simulink model "generic_src"  (Simulink 10.3)
settings: Solver=ode45  StartTime=0.0  StopTime=inf  RelTol=1e-3  EnableMultiTasking=on
undefined symbols (not defined in the file or in its folder): Area_Front, Area_Rear, ay_max_off, ay_max_on, ay_per_mu_max_off, ay_per_mu_max_on, Brake_ratio, brake_valve_ctrl_kP, cat1mode1_higher, cat1mode1_lower, cat1mode2_higher, cat1mode2_lower, cat1mode3_higher, cat1mode3_lower, cat2mode1_higher, cat2mode1_lower, cat2mode2_higher, cat2mode2_lower, cat2mode3_higher, cat2mode3_lower, delta_vel, diff_lock_fac, diff_lock_off, diff_lock_on, ESP_ctrl_kD, ESP_ctrl_kI, ESP_ctrl_kP, ESP_ctrl_restore_kI, ESP_min_throttle_fac, f_ax, f_slip, g, higherlimit_highvel, higherlimit_lowvel, highervel_fac, highervelocity_fac, InitialConditionForIntegrator, limit_acc, limit_selectlow, limit_starting, limit_vdiff, locktime_throttle, lowerlimit_highvel, lowerlimit_lowvel, lowervel_fac, lowervelocity_fac, min_throttle, MPS2KMPH, MSR_ctrl_kD, MSR_ctrl_kI, MSR_ctrl_kP, MSR_min_throttle_fac, PID_kP_sideslip, PID_kP_yawrate, RADpS2RpM, rBrake, RpM2RADpS, SH_SL_switch, sideslip_vel_corr, sidesplip_deviation_max ... (+35)
libraries: CarMaker4SL x137, simulink x57, simulink_extras x6
(part 3 of 12)

== system generic_src/CarMaker/IPG Vehicle/PowerTrain/PTControl Example/PTC GearBoxOut ==
  GearBoxOut GearNoTrg : Inport
  Bus Assignment1 : BusAssignment  AssignedSignals=PTC GearboxOut0 GearNoTrg
  BusCreator : BusCreator  Inputs=12
  CreateBus PTC GearboxOut0 : Subsystem
  CreateBus PTC GearboxOut1 : Subsystem
  CreateBus PTC GearboxOut10 : Subsystem
  CreateBus PTC GearboxOut11 : Subsystem
  CreateBus PTC GearboxOut2 : Subsystem
  CreateBus PTC GearboxOut3 : Subsystem
  CreateBus PTC GearboxOut4 : Subsystem
  CreateBus PTC GearboxOut5 : Subsystem
  CreateBus PTC GearboxOut6 : Subsystem
  CreateBus PTC GearboxOut7 : Subsystem
  CreateBus PTC GearboxOut8 : Subsystem
  CreateBus PTC GearboxOut9 : Subsystem
  Ground PTC GearboxOut{0..11} (12 alike) : Ground
  PTC GearboxOut : Outport
  wires:
  GearBoxOut GearNoTrg/1 -> Bus Assignment1/2
  Ground PTC GearboxOut0/1 -> CreateBus PTC GearboxOut0/1(In)
  CreateBus PTC GearboxOut0/1(Out) -> Bus Assignment1/1
  Ground PTC GearboxOut3/1 -> CreateBus PTC GearboxOut3/1(In)
  Ground PTC GearboxOut2/1 -> CreateBus PTC GearboxOut2/1(In)
  Ground PTC GearboxOut1/1 -> CreateBus PTC GearboxOut1/1(In)
  Ground PTC GearboxOut4/1 -> CreateBus PTC GearboxOut4/1(In)
  Ground PTC GearboxOut5/1 -> CreateBus PTC GearboxOut5/1(In)
  Ground PTC GearboxOut6/1 -> CreateBus PTC GearboxOut6/1(In)
  Ground PTC GearboxOut7/1 -> CreateBus PTC GearboxOut7/1(In)
  Ground PTC GearboxOut8/1 -> CreateBus PTC GearboxOut8/1(In)
  Ground PTC GearboxOut9/1 -> CreateBus PTC GearboxOut9/1(In)
  Ground PTC GearboxOut10/1 -> CreateBus PTC GearboxOut10/1(In)
  Ground PTC GearboxOut11/1 -> CreateBus PTC GearboxOut11/1(In)
  Bus Assignment1/1 -> BusCreator/1  "PTC GearBoxOut0"
  CreateBus PTC GearboxOut1/1(Out) -> BusCreator/2  "PTC GearBoxOut1"
  CreateBus PTC GearboxOut2/1(Out) -> BusCreator/3  "PTC GearBoxOut2"
  CreateBus PTC GearboxOut3/1(Out) -> BusCreator/4  "PTC GearBoxOut3"
  CreateBus PTC GearboxOut4/1(Out) -> BusCreator/5  "PTC GearBoxOut4"
  CreateBus PTC GearboxOut5/1(Out) -> BusCreator/6  "PTC GearBoxOut5"
  CreateBus PTC GearboxOut6/1(Out) -> BusCreator/7  "PTC GearBoxOut6"
  CreateBus PTC GearboxOut7/1(Out) -> BusCreator/8  "PTC GearBoxOut7"
  CreateBus PTC GearboxOut8/1(Out) -> BusCreator/9  "PTC GearBoxOut8"
  CreateBus PTC GearboxOut9/1(Out) -> BusCreator/10  "PTC GearBoxOut9"
  CreateBus PTC GearboxOut10/1(Out) -> BusCreator/11  "PTC GearBoxOut10"
  CreateBus PTC GearboxOut11/1(Out) -> BusCreator/12  "PTC GearBoxOut11"
  BusCreator/1 -> PTC GearboxOut/1  "PTC GearboxOut"

== system generic_src/CarMaker/IPG Vehicle/PowerTrain/PTControl Example/PTC MotorOut ==
  BusCreator : BusCreator  Inputs=12
  CreateBus PTC MotorOut0 : Subsystem
  CreateBus PTC MotorOut1 : Subsystem
  CreateBus PTC MotorOut10 : Subsystem
  CreateBus PTC MotorOut11 : Subsystem
  CreateBus PTC MotorOut2 : Subsystem
  CreateBus PTC MotorOut3 : Subsystem
  CreateBus PTC MotorOut4 : Subsystem
  CreateBus PTC MotorOut5 : Subsystem
  CreateBus PTC MotorOut6 : Subsystem
  CreateBus PTC MotorOut7 : Subsystem
  CreateBus PTC MotorOut8 : Subsystem
  CreateBus PTC MotorOut9 : Subsystem
  Ground PTC MotorOut{0..11} (12 alike) : Ground
  PTC MotorOut : Outport
  wires:
  CreateBus PTC MotorOut0/1(Out) -> BusCreator/1  "PTC MotorOut0"
  Ground PTC MotorOut0/1 -> CreateBus PTC MotorOut0/1(In)
  Ground PTC MotorOut3/1 -> CreateBus PTC MotorOut3/1(In)
  Ground PTC MotorOut1/1 -> CreateBus PTC MotorOut1/1(In)
  CreateBus PTC MotorOut1/1(Out) -> BusCreator/2  "PTC MotorOut1"
  Ground PTC MotorOut4/1 -> CreateBus PTC MotorOut4/1(In)
  Ground PTC MotorOut2/1 -> CreateBus PTC MotorOut2/1(In)
  CreateBus PTC MotorOut2/1(Out) -> BusCreator/3  "PTC MotorOut2"
  Ground PTC MotorOut5/1 -> CreateBus PTC MotorOut5/1(In)
  Ground PTC MotorOut6/1 -> CreateBus PTC MotorOut6/1(In)
  Ground PTC MotorOut7/1 -> CreateBus PTC MotorOut7/1(In)
  Ground PTC MotorOut8/1 -> CreateBus PTC MotorOut8/1(In)
  Ground PTC MotorOut9/1 -> CreateBus PTC MotorOut9/1(In)
  Ground PTC MotorOut10/1 -> CreateBus PTC MotorOut10/1(In)
  Ground PTC MotorOut11/1 -> CreateBus PTC MotorOut11/1(In)
  CreateBus PTC MotorOut4/1(Out) -> BusCreator/5  "PTC MotorOut4"
  CreateBus PTC MotorOut5/1(Out) -> BusCreator/6  "PTC MotorOut5"
  CreateBus PTC MotorOut6/1(Out) -> BusCreator/7  "PTC MotorOut6"
  CreateBus PTC MotorOut7/1(Out) -> BusCreator/8  "PTC MotorOut7"
  CreateBus PTC MotorOut8/1(Out) -> BusCreator/9  "PTC MotorOut8"
  CreateBus PTC MotorOut9/1(Out) -> BusCreator/10  "PTC MotorOut9"
  CreateBus PTC MotorOut10/1(Out) -> BusCreator/11  "PTC MotorOut10"
  CreateBus PTC MotorOut11/1(Out) -> BusCreator/12  "PTC MotorOut11"
  CreateBus PTC MotorOut3/1(Out) -> BusCreator/4  "PTC MotorOut3"
  BusCreator/1 -> PTC MotorOut/1  "CreateBus PTC MotorOut"

== system generic_src/CarMaker/IPG Vehicle/PowerTrain/PTControl Example/PTControl Example ==
  note: Minimalistic PTControl example model, that only works with
      | the 'Generic' powertrain and the 'Manual' gearbox.
  EngineIn : Inport
  VhclCtrl.PT : Inport  Port=2
  Bus Selector : BusSelector  OutputSignals=VhclCtrl Key,VhclCtrl Gas,VhclCtrl Clutch,VhclCtrl GearNo
  Bus Selector1 : BusSelector  OutputSignals=PTC EngineIn.PTC EngineIn Engine_on
  Engine : Subsystem
  ISG : Subsystem
  PTC : Subsystem
  PTC MiscOut : Outport  VectorParamsAs1DForOutWhenUnconnected=off
  EngineOut : Outport  Port=2  VectorParamsAs1DForOutWhenUnconnected=off
  ISGOut : Outport  Port=3  VectorParamsAs1DForOutWhenUnconnected=off
  ClutchOut Pos : Outport  Port=4  VectorParamsAs1DForOutWhenUnconnected=off
  GearBoxOut GearNoTrg : Outport  Port=5  VectorParamsAs1DForOutWhenUnconnected=off
  wires:
  VhclCtrl.PT/1 -> Bus Selector/1
  EngineIn/1 -> Bus Selector1/1
  Engine/1(EngineOut) -> EngineOut/1
  Bus Selector1/1 -> Engine/2(Engine_on), PTC/2(Engine_on)  "<PTC EngineIn Engine_on>"
  Bus Selector/2 -> Engine/1(Gas)  "<VhclCtrl Gas>"
  ISG/1(ISGOut) -> ISGOut/1
  PTC/1(PTC MiscOut) -> PTC MiscOut/1
  Bus Selector/4 -> GearBoxOut GearNoTrg/1  "<VhclCtrl GearNo>"
  Bus Selector/3 -> ClutchOut Pos/1  "<VhclCtrl Clutch>"
  Bus Selector/1 -> PTC/1(Key), ISG/1(Key)  "<VhclCtrl Key>"

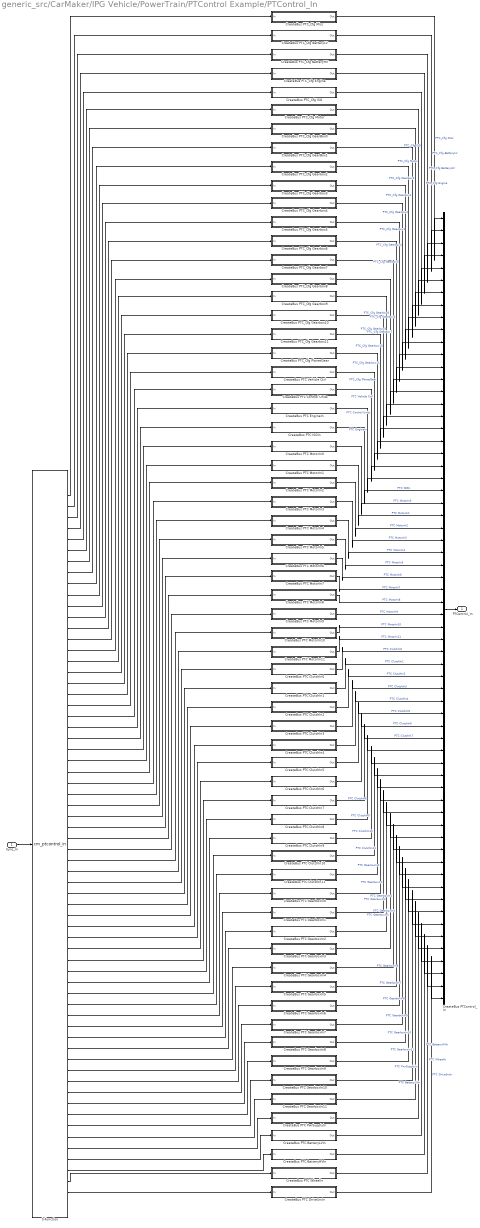
== system generic_src/CarMaker/IPG Vehicle/PowerTrain/PTControl Example/PTControl_In ==
  Sync_In : Inport
  CreateBus PTC BatteryHVIn : Subsystem
  CreateBus PTC BatteryLVIn : Subsystem
  CreateBus PTC ClutchIn0 : Subsystem
  CreateBus PTC ClutchIn1 : Subsystem
  CreateBus PTC ClutchIn10 : Subsystem
  CreateBus PTC ClutchIn11 : Subsystem
  CreateBus PTC ClutchIn2 : Subsystem
  CreateBus PTC ClutchIn3 : Subsystem
  CreateBus PTC ClutchIn4 : Subsystem
  CreateBus PTC ClutchIn5 : Subsystem
  CreateBus PTC ClutchIn6 : Subsystem
  CreateBus PTC ClutchIn7 : Subsystem
  CreateBus PTC ClutchIn8 : Subsystem
  CreateBus PTC ClutchIn9 : Subsystem
  CreateBus PTC Control Units : Subsystem
  CreateBus PTC DriveSrcIn : Subsystem
  CreateBus PTC EngineIn : Subsystem
  CreateBus PTC GearboxIn0 : Subsystem
  CreateBus PTC GearboxIn1 : Subsystem
  CreateBus PTC GearboxIn10 : Subsystem
  CreateBus PTC GearboxIn11 : Subsystem
  CreateBus PTC GearboxIn2 : Subsystem
  CreateBus PTC GearboxIn3 : Subsystem
  CreateBus PTC GearboxIn4 : Subsystem
  CreateBus PTC GearboxIn5 : Subsystem
  CreateBus PTC GearboxIn6 : Subsystem
  CreateBus PTC GearboxIn7 : Subsystem
  CreateBus PTC GearboxIn8 : Subsystem
  CreateBus PTC GearboxIn9 : Subsystem
  CreateBus PTC ISGIn : Subsystem
  CreateBus PTC MotorIn0 : Subsystem
  CreateBus PTC MotorIn1 : Subsystem
  CreateBus PTC MotorIn10 : Subsystem
  CreateBus PTC MotorIn11 : Subsystem
  CreateBus PTC MotorIn2 : Subsystem
  CreateBus PTC MotorIn3 : Subsystem
  CreateBus PTC MotorIn4 : Subsystem
  CreateBus PTC MotorIn5 : Subsystem
  CreateBus PTC MotorIn6 : Subsystem
  CreateBus PTC MotorIn7 : Subsystem
  CreateBus PTC MotorIn8 : Subsystem
  CreateBus PTC MotorIn9 : Subsystem
  CreateBus PTC PwrSupplyIn : Subsystem
  CreateBus PTC Vehicle Ctrl : Subsystem
  CreateBus PTC WheelIn : Subsystem
  CreateBus PTC_Cfg BatteryHV : Subsystem
  CreateBus PTC_Cfg BatteryLV : Subsystem
  CreateBus PTC_Cfg Engine : Subsystem
  CreateBus PTC_Cfg GearBox0 : Subsystem
  CreateBus PTC_Cfg GearBox1 : Subsystem
  CreateBus PTC_Cfg Gearbox10 : Subsystem
  CreateBus PTC_Cfg Gearbox11 : Subsystem
  CreateBus PTC_Cfg Gearbox2 : Subsystem
  CreateBus PTC_Cfg Gearbox3 : Subsystem
  CreateBus PTC_Cfg Gearbox4 : Subsystem
  CreateBus PTC_Cfg Gearbox5 : Subsystem
  CreateBus PTC_Cfg Gearbox6 : Subsystem
  CreateBus PTC_Cfg Gearbox7 : Subsystem
  CreateBus PTC_Cfg Gearbox8 : Subsystem
  CreateBus PTC_Cfg Gearbox9 : Subsystem
  CreateBus PTC_Cfg ISG : Subsystem
  CreateBus PTC_Cfg Misc : Subsystem
  CreateBus PTC_Cfg Motor : Subsystem
  CreateBus PTC_Cfg PlanetGear : Subsystem
  CreateBus PTControl_In : BusCreator  Inputs=64
  S-Function : S-Function  FunctionName=cm_ptcontrol_in  SFunctionDeploymentMode=off  EnableBusSupport=off
  PTControl_In : Outport  VectorParamsAs1DForOutWhenUnconnected=off
  wires:
  CreateBus PTControl_In/1 -> PTControl_In/1
  Sync_In/1 -> S-Function/1
  S-Function/2 -> CreateBus PTC_Cfg BatteryLV/1(In)
  CreateBus PTC_Cfg Misc/1(Out) -> CreateBus PTControl_In/1  "PTC_Cfg Misc"
  S-Function/1 -> CreateBus PTC_Cfg Misc/1(In)
  CreateBus PTC_Cfg Motor/1(Out) -> CreateBus PTControl_In/6  "PTC_Cfg Motor"
  CreateBus PTC_Cfg Gearbox2/1(Out) -> CreateBus PTControl_In/9  "PTC_Cfg Gearbox2"
  S-Function/4 -> CreateBus PTC_Cfg Engine/1(In)
  S-Function/3 -> CreateBus PTC_Cfg BatteryHV/1(In)
  S-Function/7 -> CreateBus PTC_Cfg GearBox0/1(In)
  S-Function/14 -> CreateBus PTC_Cfg Gearbox7/1(In)
  S-Function/15 -> CreateBus PTC_Cfg Gearbox8/1(In)
  S-Function/17 -> CreateBus PTC_Cfg Gearbox10/1(In)
  S-Function/18 -> CreateBus PTC_Cfg Gearbox11/1(In)
  CreateBus PTC_Cfg GearBox1/1(Out) -> CreateBus PTControl_In/8  "PTC_Cfg Gearbox1"
  CreateBus PTC_Cfg Gearbox4/1(Out) -> CreateBus PTControl_In/11  "PTC_Cfg Gearbox4"
  CreateBus PTC_Cfg Gearbox5/1(Out) -> CreateBus PTControl_In/12  "PTC_Cfg Gearbox5"
  CreateBus PTC_Cfg Gearbox6/1(Out) -> CreateBus PTControl_In/13  "PTC_Cfg Gearbox6"
  CreateBus PTC_Cfg Gearbox7/1(Out) -> CreateBus PTControl_In/14  "PTC_Cfg Gearbox7"
  CreateBus PTC GearboxIn6/1(Out) -> CreateBus PTControl_In/54  "PTC GearboxIn6"
  CreateBus PTC ClutchIn6/1(Out) -> CreateBus PTControl_In/42  "PTC ClutchIn6"
  CreateBus PTC GearboxIn5/1(Out) -> CreateBus PTControl_In/53  "PTC GearboxIn5"
  CreateBus PTC GearboxIn9/1(Out) -> CreateBus PTControl_In/57  "PTC GearboxIn9"
  CreateBus PTC ClutchIn8/1(Out) -> CreateBus PTControl_In/44  "PTC ClutchIn8"
  S-Function/32 -> CreateBus PTC MotorIn8/1(In)
  CreateBus PTC MotorIn0/1(Out) -> CreateBus PTControl_In/24  "PTC MotorIn0"
  S-Function/8 -> CreateBus PTC_Cfg GearBox1/1(In)
  S-Function/46 -> CreateBus PTC ClutchIn10/1(In)
  S-Function/61 -> CreateBus PTC BatteryLVIn/1(In)
  S-Function/11 -> CreateBus PTC_Cfg Gearbox4/1(In)
  S-Function/37 -> CreateBus PTC ClutchIn1/1(In)
  S-Function/50 -> CreateBus PTC GearboxIn2/1(In)
  CreateBus PTC WheelIn/1(Out) -> CreateBus PTControl_In/63  "PTC WheelIn"
  S-Function/24 -> CreateBus PTC MotorIn0/1(In)
  CreateBus PTC_Cfg Gearbox3/1(Out) -> CreateBus PTControl_In/10  "PTC_Cfg Gearbox3"
  S-Function/51 -> CreateBus PTC GearboxIn3/1(In)
  S-Function/56 -> CreateBus PTC GearboxIn8/1(In)
  CreateBus PTC GearboxIn3/1(Out) -> CreateBus PTControl_In/51  "PTC GearboxIn3"
  CreateBus PTC MotorIn1/1(Out) -> CreateBus PTControl_In/25  "PTC MotorIn1"
  S-Function/10 -> CreateBus PTC_Cfg Gearbox3/1(In)
  CreateBus PTC DriveSrcIn/1(Out) -> CreateBus PTControl_In/64  "PTC DriveSrcIn"
  CreateBus PTC ISGIn/1(Out) -> CreateBus PTControl_In/23  "PTC ISGIn"
  CreateBus PTC ClutchIn11/1(Out) -> CreateBus PTControl_In/47  "PTC ClutchIn11"
  S-Function/20 -> CreateBus PTC Vehicle Ctrl/1(In)
  S-Function/47 -> CreateBus PTC ClutchIn11/1(In)
  S-Function/64 -> CreateBus PTC DriveSrcIn/1(In)
  CreateBus PTC ClutchIn10/1(Out) -> CreateBus PTControl_In/46  "PTC ClutchIn10"
  CreateBus PTC GearboxIn2/1(Out) -> CreateBus PTControl_In/50  "PTC GearboxIn2"
  CreateBus PTC GearboxIn0/1(Out) -> CreateBus PTControl_In/48  "PTC GearboxIn0"
  S-Function/16 -> CreateBus PTC_Cfg Gearbox9/1(In)
  S-Function/25 -> CreateBus PTC MotorIn1/1(In)
  S-Function/63 -> CreateBus PTC WheelIn/1(In)
  CreateBus PTC GearboxIn1/1(Out) -> CreateBus PTControl_In/49  "PTC GearboxIn1"
  S-Function/33 -> CreateBus PTC MotorIn9/1(In)
  CreateBus PTC BatteryLVIn/1(Out) -> CreateBus PTControl_In/61  "PTC BatteryLVIn"
  S-Function/58 -> CreateBus PTC GearboxIn10/1(In)
  S-Function/41 -> CreateBus PTC ClutchIn5/1(In)
  S-Function/5 -> CreateBus PTC_Cfg ISG/1(In)
  S-Function/44 -> CreateBus PTC ClutchIn8/1(In)
  S-Function/45 -> CreateBus PTC ClutchIn9/1(In)
  CreateBus PTC GearboxIn11/1(Out) -> CreateBus PTControl_In/59  "PTC GearboxIn11"
  S-Function/9 -> CreateBus PTC_Cfg Gearbox2/1(In)
  S-Function/35 -> CreateBus PTC MotorIn11/1(In)
  S-Function/19 -> CreateBus PTC_Cfg PlanetGear/1(In)
  CreateBus PTC GearboxIn8/1(Out) -> CreateBus PTControl_In/56  "PTC GearboxIn8"
  S-Function/36 -> CreateBus PTC ClutchIn0/1(In)
  S-Function/53 -> CreateBus PTC GearboxIn5/1(In)
  CreateBus PTC GearboxIn10/1(Out) -> CreateBus PTControl_In/58  "PTC GearboxIn10"
  S-Function/6 -> CreateBus PTC_Cfg Motor/1(In)
  CreateBus PTC PwrSupplyIn/1(Out) -> CreateBus PTControl_In/60  "PTC PwrSupplyIn"
  S-Function/43 -> CreateBus PTC ClutchIn7/1(In)
  CreateBus PTC_Cfg BatteryLV/1(Out) -> CreateBus PTControl_In/2  "PTC_Cfg BatteryLV"
  CreateBus PTC ClutchIn1/1(Out) -> CreateBus PTControl_In/37  "PTC ClutchIn1"
  S-Function/26 -> CreateBus PTC MotorIn2/1(In)
  CreateBus PTC_Cfg PlanetGear/1(Out) -> CreateBus PTControl_In/19  "PTC_Cfg PlanetGear"
  CreateBus PTC_Cfg Gearbox10/1(Out) -> CreateBus PTControl_In/17  "PTC_Cfg Gearbox10"
  CreateBus PTC ClutchIn7/1(Out) -> CreateBus PTControl_In/43  "PTC ClutchIn7"
  S-Function/54 -> CreateBus PTC GearboxIn6/1(In)
  S-Function/29 -> CreateBus PTC MotorIn5/1(In)
  CreateBus PTC_Cfg BatteryHV/1(Out) -> CreateBus PTControl_In/3  "PTC_Cfg BatteryHV"
  S-Function/13 -> CreateBus PTC_Cfg Gearbox6/1(In)
  CreateBus PTC ClutchIn9/1(Out) -> CreateBus PTControl_In/45  "PTC ClutchIn9"
  CreateBus PTC GearboxIn4/1(Out) -> CreateBus PTControl_In/52  "PTC GearboxIn4"
  S-Function/57 -> CreateBus PTC GearboxIn9/1(In)
  CreateBus PTC GearboxIn7/1(Out) -> CreateBus PTControl_In/55  "PTC GearboxIn7"
  S-Function/60 -> CreateBus PTC PwrSupplyIn/1(In)
  CreateBus PTC BatteryHVIn/1(Out) -> CreateBus PTControl_In/62  "PTC BatteryHVIn"
  S-Function/49 -> CreateBus PTC GearboxIn1/1(In)
  S-Function/55 -> CreateBus PTC GearboxIn7/1(In)
  S-Function/21 -> CreateBus PTC Control Units/1(In)
  CreateBus PTC ClutchIn5/1(Out) -> CreateBus PTControl_In/41  "PTC ClutchIn5"
  CreateBus PTC ClutchIn4/1(Out) -> CreateBus PTControl_In/40  "PTC ClutchIn4"
  S-Function/38 -> CreateBus PTC ClutchIn2/1(In)
  CreateBus PTC Control Units/1(Out) -> CreateBus PTControl_In/21  "PTC Control Units"
  S-Function/40 -> CreateBus PTC ClutchIn4/1(In)
  CreateBus PTC MotorIn11/1(Out) -> CreateBus PTControl_In/35  "PTC MotorIn11"
  CreateBus PTC ClutchIn3/1(Out) -> CreateBus PTControl_In/39  "PTC ClutchIn3"
  S-Function/39 -> CreateBus PTC ClutchIn3/1(In)
  CreateBus PTC MotorIn2/1(Out) -> CreateBus PTControl_In/26  "PTC MotorIn2"
  CreateBus PTC ClutchIn2/1(Out) -> CreateBus PTControl_In/38  "PTC ClutchIn2"
  CreateBus PTC_Cfg ISG/1(Out) -> CreateBus PTControl_In/5  "PTC_Cfg ISG"
  CreateBus PTC ClutchIn0/1(Out) -> CreateBus PTControl_In/36  "PTC ClutchIn0"
  S-Function/52 -> CreateBus PTC GearboxIn4/1(In)
  CreateBus PTC EngineIn/1(Out) -> CreateBus PTControl_In/22  "PTC EngineIn"
  CreateBus PTC_Cfg GearBox0/1(Out) -> CreateBus PTControl_In/7  "PTC_Cfg Gearbox0"
  S-Function/42 -> CreateBus PTC ClutchIn6/1(In)
  S-Function/34 -> CreateBus PTC MotorIn10/1(In)
  CreateBus PTC MotorIn9/1(Out) -> CreateBus PTControl_In/33  "PTC MotorIn9"
  S-Function/30 -> CreateBus PTC MotorIn6/1(In)
  S-Function/12 -> CreateBus PTC_Cfg Gearbox5/1(In)
  CreateBus PTC MotorIn8/1(Out) -> CreateBus PTControl_In/32  "PTC MotorIn8"
  CreateBus PTC MotorIn7/1(Out) -> CreateBus PTControl_In/31  "PTC MotorIn7"
  S-Function/31 -> CreateBus PTC MotorIn7/1(In)
  CreateBus PTC MotorIn6/1(Out) -> CreateBus PTControl_In/30  "PTC MotorIn6"
  CreateBus PTC MotorIn4/1(Out) -> CreateBus PTControl_In/28  "PTC MotorIn4"
  S-Function/62 -> CreateBus PTC BatteryHVIn/1(In)
  S-Function/27 -> CreateBus PTC MotorIn3/1(In)
  S-Function/28 -> CreateBus PTC MotorIn4/1(In)
  CreateBus PTC MotorIn5/1(Out) -> CreateBus PTControl_In/29  "PTC MotorIn5"
  CreateBus PTC MotorIn3/1(Out) -> CreateBus PTControl_In/27  "PTC MotorIn3"
  S-Function/23 -> CreateBus PTC ISGIn/1(In)
  S-Function/22 -> CreateBus PTC EngineIn/1(In)
  CreateBus PTC_Cfg Engine/1(Out) -> CreateBus PTControl_In/4  "PTC_Cfg Engine"
  S-Function/48 -> CreateBus PTC GearboxIn0/1(In)
  S-Function/59 -> CreateBus PTC GearboxIn11/1(In)
  CreateBus PTC Vehicle Ctrl/1(Out) -> CreateBus PTControl_In/20  "PTC Vehicle Ctrl"
  CreateBus PTC MotorIn10/1(Out) -> CreateBus PTControl_In/34  "PTC MotorIn10"
  CreateBus PTC_Cfg Gearbox11/1(Out) -> CreateBus PTControl_In/18  "PTC_Cfg Gearbox11"
  CreateBus PTC_Cfg Gearbox9/1(Out) -> CreateBus PTControl_In/16  "PTC_Cfg Gearbox9"
  CreateBus PTC_Cfg Gearbox8/1(Out) -> CreateBus PTControl_In/15  "PTC_Cfg Gearbox8"

== system generic_src/CarMaker/IPG Vehicle/PowerTrain/PTControl Example/PTControl_Out ==
  PTC MiscOut : Inport
  PTC EngineOut : Inport  Port=2
  PTC ISGOut : Inport  Port=3
  PTC MotorOut : Inport  Port=4
  PTC ClutchOut : Inport  Port=5
  PTC GearboxOut : Inport  Port=6
  PTC PwrSupplyOut : Inport  Port=7
  PTC BattLV_Out : Inport  Port=8
  PTC BattHV_Out : Inport  Port=9
  PTC WheelOut : Inport  Port=10
  Bus Selector1 : BusSelector  OutputSignals=PTC MotorOut0,PTC MotorOut1,PTC MotorOut2,PTC MotorOut3,PTC MotorOut4,PTC MotorOut5,PTC MotorOut6,PTC MotorOut7,PTC MotorOut8,PTC MotorOut9,PTC MotorOut10,PTC MotorOut11
  Bus Selector2 : BusSelector  OutputSignals=PTC ClutchOut0,PTC ClutchOut1,PTC ClutchOut2,PTC ClutchOut3,PTC ClutchOut4,PTC ClutchOut5,PTC ClutchOut6,PTC ClutchOut7,PTC ClutchOut8,PTC ClutchOut9,PTC ClutchOut10,PTC ClutchOut11
  Bus Selector3 : BusSelector  OutputSignals=PTC GearBoxOut0,PTC GearBoxOut1,PTC GearBoxOut2,PTC GearBoxOut3,PTC GearBoxOut4,PTC GearBoxOut5,PTC GearBoxOut6,PTC GearBoxOut7,PTC GearBoxOut8,PTC GearBoxOut9,PTC GearBoxOut10,PTC GearBoxOut11
  PTControl_Out : S-Function  FunctionName=cm_ptcontrol_out  SFunctionDeploymentMode=off  EnableBusSupport=off
  wires:
  PTC MotorOut/1 -> Bus Selector1/1
  PTC ISGOut/1 -> PTControl_Out/3
  PTC EngineOut/1 -> PTControl_Out/2
  PTC MiscOut/1 -> PTControl_Out/1
  Bus Selector1/1 -> PTControl_Out/4  "<PTC MotorOut0>"
  Bus Selector1/2 -> PTControl_Out/5  "<PTC MotorOut1>"
  Bus Selector1/3 -> PTControl_Out/6  "<PTC MotorOut2>"
  Bus Selector1/4 -> PTControl_Out/7  "<PTC MotorOut3>"
  Bus Selector1/5 -> PTControl_Out/8  "<PTC MotorOut4>"
  Bus Selector1/6 -> PTControl_Out/9  "<PTC MotorOut5>"
  Bus Selector1/7 -> PTControl_Out/10  "<PTC MotorOut6>"
  Bus Selector1/8 -> PTControl_Out/11  "<PTC MotorOut7>"
  Bus Selector1/9 -> PTControl_Out/12  "<PTC MotorOut8>"
  Bus Selector1/10 -> PTControl_Out/13  "<PTC MotorOut9>"
  Bus Selector1/11 -> PTControl_Out/14  "<PTC MotorOut10>"
  Bus Selector1/12 -> PTControl_Out/15  "<PTC MotorOut11>"
  PTC ClutchOut/1 -> Bus Selector2/1
  Bus Selector2/1 -> PTControl_Out/16  "<PTC ClutchOut0>"
  Bus Selector2/2 -> PTControl_Out/17  "<PTC ClutchOut1>"
  Bus Selector2/3 -> PTControl_Out/18  "<PTC ClutchOut2>"
  Bus Selector2/4 -> PTControl_Out/19  "<PTC ClutchOut3>"
  Bus Selector2/5 -> PTControl_Out/20  "<PTC ClutchOut4>"
  Bus Selector2/6 -> PTControl_Out/21  "<PTC ClutchOut5>"
  Bus Selector2/7 -> PTControl_Out/22  "<PTC ClutchOut6>"
  Bus Selector2/8 -> PTControl_Out/23  "<PTC ClutchOut7>"
  Bus Selector2/9 -> PTControl_Out/24  "<PTC ClutchOut8>"
  Bus Selector2/10 -> PTControl_Out/25  "<PTC ClutchOut9>"
  Bus Selector2/11 -> PTControl_Out/26  "<PTC ClutchOut10>"
  Bus Selector2/12 -> PTControl_Out/27  "<PTC ClutchOut11>"
  PTC GearboxOut/1 -> Bus Selector3/1
  Bus Selector3/1 -> PTControl_Out/28  "<PTC GearBoxOut0>"
  Bus Selector3/2 -> PTControl_Out/29  "<PTC GearBoxOut1>"
  Bus Selector3/3 -> PTControl_Out/30  "<PTC GearBoxOut2>"
  Bus Selector3/4 -> PTControl_Out/31  "<PTC GearBoxOut3>"
  Bus Selector3/5 -> PTControl_Out/32  "<PTC GearBoxOut4>"
  Bus Selector3/6 -> PTControl_Out/33  "<PTC GearBoxOut5>"
  Bus Selector3/7 -> PTControl_Out/34  "<PTC GearBoxOut6>"
  Bus Selector3/8 -> PTControl_Out/35  "<PTC GearBoxOut7>"
  Bus Selector3/9 -> PTControl_Out/36  "<PTC GearBoxOut8>"
  Bus Selector3/10 -> PTControl_Out/37  "<PTC GearBoxOut9>"
  Bus Selector3/11 -> PTControl_Out/38  "<PTC GearBoxOut10>"
  Bus Selector3/12 -> PTControl_Out/39  "<PTC GearBoxOut11>"
  PTC PwrSupplyOut/1 -> PTControl_Out/40
  PTC BattLV_Out/1 -> PTControl_Out/41
  PTC BattHV_Out/1 -> PTControl_Out/42
  PTC WheelOut/1 -> PTControl_Out/43

== system generic_src/CarMaker/IPG Vehicle/PowerTrain/TCU Example/CreateBus TCU Status ==
  In : Inport
  BusCreator : BusCreator  Inputs=1
  Demux : Demux  Outputs=1
      settings: DisplayOption=none
  Out : Outport  VectorParamsAs1DForOutWhenUnconnected=off
  wires:
  Demux/1 -> BusCreator/1  "TCU_Out Status"
  BusCreator/1 -> Out/1
  In/1 -> Demux/1

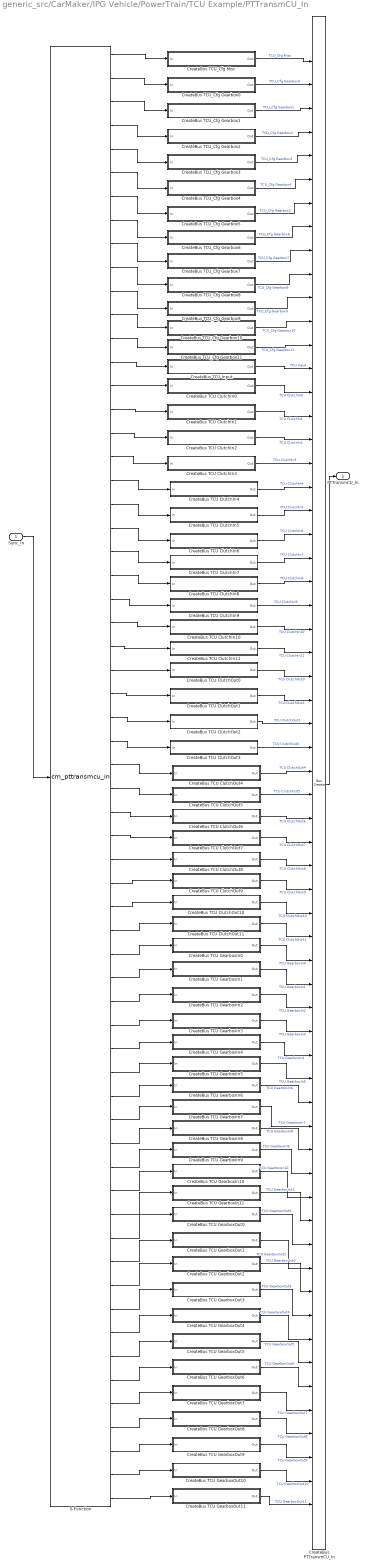
== system generic_src/CarMaker/IPG Vehicle/PowerTrain/TCU Example/PTTransmCU_In ==
  Sync_In : Inport
  CreateBus PTTransmCU_In : BusCreator  Inputs=62
  CreateBus TCU ClutchIn0 : Subsystem
  CreateBus TCU ClutchIn1 : Subsystem
  CreateBus TCU ClutchIn10 : Subsystem
  CreateBus TCU ClutchIn11 : Subsystem
  CreateBus TCU ClutchIn2 : Subsystem
  CreateBus TCU ClutchIn3 : Subsystem
  CreateBus TCU ClutchIn4 : Subsystem
  CreateBus TCU ClutchIn5 : Subsystem
  CreateBus TCU ClutchIn6 : Subsystem
  CreateBus TCU ClutchIn7 : Subsystem
  CreateBus TCU ClutchIn8 : Subsystem
  CreateBus TCU ClutchIn9 : Subsystem
  CreateBus TCU ClutchOut0 : Subsystem
  CreateBus TCU ClutchOut1 : Subsystem
  CreateBus TCU ClutchOut10 : Subsystem
  CreateBus TCU ClutchOut11 : Subsystem
  CreateBus TCU ClutchOut2 : Subsystem
  CreateBus TCU ClutchOut3 : Subsystem
  CreateBus TCU ClutchOut4 : Subsystem
  CreateBus TCU ClutchOut5 : Subsystem
  CreateBus TCU ClutchOut6 : Subsystem
  CreateBus TCU ClutchOut7 : Subsystem
  CreateBus TCU ClutchOut8 : Subsystem
  CreateBus TCU ClutchOut9 : Subsystem
  CreateBus TCU GearboxIn0 : Subsystem
  CreateBus TCU GearboxIn1 : Subsystem
  CreateBus TCU GearboxIn10 : Subsystem
  CreateBus TCU GearboxIn11 : Subsystem
  CreateBus TCU GearboxIn2 : Subsystem
  CreateBus TCU GearboxIn3 : Subsystem
  CreateBus TCU GearboxIn4 : Subsystem
  CreateBus TCU GearboxIn5 : Subsystem
  CreateBus TCU GearboxIn6 : Subsystem
  CreateBus TCU GearboxIn7 : Subsystem
  CreateBus TCU GearboxIn8 : Subsystem
  CreateBus TCU GearboxIn9 : Subsystem
  CreateBus TCU GearboxOut0 : Subsystem
  CreateBus TCU GearboxOut1 : Subsystem
  CreateBus TCU GearboxOut10 : Subsystem
  CreateBus TCU GearboxOut11 : Subsystem
  CreateBus TCU GearboxOut2 : Subsystem
  CreateBus TCU GearboxOut3 : Subsystem
  CreateBus TCU GearboxOut4 : Subsystem
  CreateBus TCU GearboxOut5 : Subsystem
  CreateBus TCU GearboxOut6 : Subsystem
  CreateBus TCU GearboxOut7 : Subsystem
  CreateBus TCU GearboxOut8 : Subsystem
  CreateBus TCU GearboxOut9 : Subsystem
  CreateBus TCU Input : Subsystem
  CreateBus TCU_Cfg Gearbox0 : Subsystem
  CreateBus TCU_Cfg Gearbox1 : Subsystem
  CreateBus TCU_Cfg Gearbox10 : Subsystem
  CreateBus TCU_Cfg Gearbox11 : Subsystem
  CreateBus TCU_Cfg Gearbox2 : Subsystem
  CreateBus TCU_Cfg Gearbox3 : Subsystem
  CreateBus TCU_Cfg Gearbox4 : Subsystem
  CreateBus TCU_Cfg Gearbox5 : Subsystem
  CreateBus TCU_Cfg Gearbox6 : Subsystem
  CreateBus TCU_Cfg Gearbox7 : Subsystem
  CreateBus TCU_Cfg Gearbox8 : Subsystem
  CreateBus TCU_Cfg Gearbox9 : Subsystem
  CreateBus TCU_Cfg Misc : Subsystem
  S-Function : S-Function  FunctionName=cm_pttransmcu_in  SFunctionDeploymentMode=off  EnableBusSupport=off
  PTTransmCU_In : Outport  VectorParamsAs1DForOutWhenUnconnected=off
  wires:
  CreateBus TCU_Cfg Gearbox3/1(Out) -> CreateBus PTTransmCU_In/5  "TCU_Cfg Gearbox3"
  CreateBus TCU_Cfg Misc/1(Out) -> CreateBus PTTransmCU_In/1  "TCU_Cfg Misc"
  S-Function/1 -> CreateBus TCU_Cfg Misc/1(In)
  CreateBus PTTransmCU_In/1 -> PTTransmCU_In/1
  S-Function/5 -> CreateBus TCU_Cfg Gearbox3/1(In)
  CreateBus TCU_Cfg Gearbox2/1(Out) -> CreateBus PTTransmCU_In/4  "TCU_Cfg Gearbox2"
  CreateBus TCU_Cfg Gearbox1/1(Out) -> CreateBus PTTransmCU_In/3  "TCU_Cfg Gearbox1"
  CreateBus TCU_Cfg Gearbox0/1(Out) -> CreateBus PTTransmCU_In/2  "TCU_Cfg Gearbox0"
  Sync_In/1 -> S-Function/1
  S-Function/2 -> CreateBus TCU_Cfg Gearbox0/1(In)
  S-Function/4 -> CreateBus TCU_Cfg Gearbox2/1(In)
  S-Function/3 -> CreateBus TCU_Cfg Gearbox1/1(In)
  S-Function/6 -> CreateBus TCU_Cfg Gearbox4/1(In)
  CreateBus TCU_Cfg Gearbox4/1(Out) -> CreateBus PTTransmCU_In/6  "TCU_Cfg Gearbox4"
  S-Function/7 -> CreateBus TCU_Cfg Gearbox5/1(In)
  CreateBus TCU_Cfg Gearbox5/1(Out) -> CreateBus PTTransmCU_In/7  "TCU_Cfg Gearbox5"
  S-Function/8 -> CreateBus TCU_Cfg Gearbox6/1(In)
  CreateBus TCU_Cfg Gearbox6/1(Out) -> CreateBus PTTransmCU_In/8  "TCU_Cfg Gearbox6"
  S-Function/9 -> CreateBus TCU_Cfg Gearbox7/1(In)
  CreateBus TCU_Cfg Gearbox7/1(Out) -> CreateBus PTTransmCU_In/9  "TCU_Cfg Gearbox7"
  S-Function/10 -> CreateBus TCU_Cfg Gearbox8/1(In)
  CreateBus TCU_Cfg Gearbox8/1(Out) -> CreateBus PTTransmCU_In/10  "TCU_Cfg Gearbox8"
  S-Function/11 -> CreateBus TCU_Cfg Gearbox9/1(In)
  S-Function/12 -> CreateBus TCU_Cfg Gearbox10/1(In)
  CreateBus TCU_Cfg Gearbox9/1(Out) -> CreateBus PTTransmCU_In/11  "TCU_Cfg Gearbox9"
  CreateBus TCU_Cfg Gearbox10/1(Out) -> CreateBus PTTransmCU_In/12  "TCU_Cfg Gearbox10"
  S-Function/13 -> CreateBus TCU_Cfg Gearbox11/1(In)
  CreateBus TCU_Cfg Gearbox11/1(Out) -> CreateBus PTTransmCU_In/13  "TCU_Cfg Gearbox11"
  S-Function/14 -> CreateBus TCU Input/1(In)
  CreateBus TCU Input/1(Out) -> CreateBus PTTransmCU_In/14  "TCU Input"
  S-Function/15 -> CreateBus TCU ClutchIn0/1(In)
  S-Function/16 -> CreateBus TCU ClutchIn1/1(In)
  S-Function/17 -> CreateBus TCU ClutchIn2/1(In)
  S-Function/18 -> CreateBus TCU ClutchIn3/1(In)
  CreateBus TCU ClutchIn1/1(Out) -> CreateBus PTTransmCU_In/16  "TCU ClutchIn1"
  CreateBus TCU ClutchIn2/1(Out) -> CreateBus PTTransmCU_In/17  "TCU ClutchIn2"
  CreateBus TCU ClutchIn3/1(Out) -> CreateBus PTTransmCU_In/18  "TCU ClutchIn3"
  S-Function/19 -> CreateBus TCU ClutchIn4/1(In)
  CreateBus TCU ClutchIn4/1(Out) -> CreateBus PTTransmCU_In/19  "TCU ClutchIn4"
  S-Function/20 -> CreateBus TCU ClutchIn5/1(In)
  CreateBus TCU ClutchIn5/1(Out) -> CreateBus PTTransmCU_In/20  "TCU ClutchIn5"
  CreateBus TCU ClutchIn6/1(Out) -> CreateBus PTTransmCU_In/21  "TCU ClutchIn6"
  S-Function/21 -> CreateBus TCU ClutchIn6/1(In)
  S-Function/22 -> CreateBus TCU ClutchIn7/1(In)
  CreateBus TCU ClutchIn7/1(Out) -> CreateBus PTTransmCU_In/22  "TCU ClutchIn7"
  S-Function/23 -> CreateBus TCU ClutchIn8/1(In)
  CreateBus TCU ClutchIn8/1(Out) -> CreateBus PTTransmCU_In/23  "TCU ClutchIn8"
  S-Function/24 -> CreateBus TCU ClutchIn9/1(In)
  CreateBus TCU ClutchIn9/1(Out) -> CreateBus PTTransmCU_In/24  "TCU ClutchIn9"
  S-Function/25 -> CreateBus TCU ClutchIn10/1(In)
  CreateBus TCU ClutchIn10/1(Out) -> CreateBus PTTransmCU_In/25  "TCU ClutchIn10"
  S-Function/26 -> CreateBus TCU ClutchIn11/1(In)
  CreateBus TCU ClutchIn11/1(Out) -> CreateBus PTTransmCU_In/26  "TCU ClutchIn11"
  S-Function/27 -> CreateBus TCU ClutchOut0/1(In)
  CreateBus TCU ClutchOut0/1(Out) -> CreateBus PTTransmCU_In/27  "TCU ClutchOut0"
  S-Function/28 -> CreateBus TCU ClutchOut1/1(In)
  CreateBus TCU ClutchOut1/1(Out) -> CreateBus PTTransmCU_In/28  "TCU ClutchOut1"
  S-Function/29 -> CreateBus TCU ClutchOut2/1(In)
  CreateBus TCU ClutchOut2/1(Out) -> CreateBus PTTransmCU_In/29  "TCU ClutchOut2"
  S-Function/30 -> CreateBus TCU ClutchOut3/1(In)
  CreateBus TCU ClutchOut3/1(Out) -> CreateBus PTTransmCU_In/30  "TCU ClutchOut3"
  CreateBus TCU ClutchOut4/1(Out) -> CreateBus PTTransmCU_In/31  "TCU ClutchOut4"
  S-Function/31 -> CreateBus TCU ClutchOut4/1(In)
  CreateBus TCU ClutchOut5/1(Out) -> CreateBus PTTransmCU_In/32  "TCU ClutchOut5"
  S-Function/32 -> CreateBus TCU ClutchOut5/1(In)
  CreateBus TCU ClutchOut6/1(Out) -> CreateBus PTTransmCU_In/33  "TCU ClutchOut6"
  S-Function/33 -> CreateBus TCU ClutchOut6/1(In)
  S-Function/34 -> CreateBus TCU ClutchOut7/1(In)
  CreateBus TCU ClutchOut7/1(Out) -> CreateBus PTTransmCU_In/34  "TCU ClutchOut7"
  S-Function/35 -> CreateBus TCU ClutchOut8/1(In)
  CreateBus TCU ClutchOut8/1(Out) -> CreateBus PTTransmCU_In/35  "TCU ClutchOut8"
  S-Function/36 -> CreateBus TCU ClutchOut9/1(In)
  CreateBus TCU ClutchOut9/1(Out) -> CreateBus PTTransmCU_In/36  "TCU ClutchOut9"
  S-Function/37 -> CreateBus TCU ClutchOut10/1(In)
  CreateBus TCU ClutchOut10/1(Out) -> CreateBus PTTransmCU_In/37  "TCU ClutchOut10"
  S-Function/38 -> CreateBus TCU ClutchOut11/1(In)
  CreateBus TCU ClutchOut11/1(Out) -> CreateBus PTTransmCU_In/38  "TCU ClutchOut11"
  S-Function/39 -> CreateBus TCU GearboxIn0/1(In)
  CreateBus TCU GearboxIn0/1(Out) -> CreateBus PTTransmCU_In/39  "TCU GearboxIn0"
  S-Function/40 -> CreateBus TCU GearboxIn1/1(In)
  CreateBus TCU GearboxIn1/1(Out) -> CreateBus PTTransmCU_In/40  "TCU GearboxIn1"
  S-Function/41 -> CreateBus TCU GearboxIn2/1(In)
  CreateBus TCU GearboxIn2/1(Out) -> CreateBus PTTransmCU_In/41  "TCU GearboxIn2"
  S-Function/42 -> CreateBus TCU GearboxIn3/1(In)
  CreateBus TCU GearboxIn3/1(Out) -> CreateBus PTTransmCU_In/42  "TCU GearboxIn3"
  S-Function/43 -> CreateBus TCU GearboxIn4/1(In)
  CreateBus TCU GearboxIn4/1(Out) -> CreateBus PTTransmCU_In/43  "TCU GearboxIn4"
  S-Function/44 -> CreateBus TCU GearboxIn5/1(In)
  CreateBus TCU GearboxIn5/1(Out) -> CreateBus PTTransmCU_In/44  "TCU GearboxIn5"
  S-Function/45 -> CreateBus TCU GearboxIn6/1(In)
  CreateBus TCU GearboxIn6/1(Out) -> CreateBus PTTransmCU_In/45  "TCU GearboxIn6"
  S-Function/46 -> CreateBus TCU GearboxIn7/1(In)
  CreateBus TCU GearboxIn7/1(Out) -> CreateBus PTTransmCU_In/46  "TCU GearboxIn7"
  S-Function/47 -> CreateBus TCU GearboxIn8/1(In)
  CreateBus TCU GearboxIn8/1(Out) -> CreateBus PTTransmCU_In/47  "TCU GearboxIn8"
  S-Function/48 -> CreateBus TCU GearboxIn9/1(In)
  CreateBus TCU GearboxIn9/1(Out) -> CreateBus PTTransmCU_In/48  "TCU GearboxIn9"
  S-Function/49 -> CreateBus TCU GearboxIn10/1(In)
  CreateBus TCU GearboxIn10/1(Out) -> CreateBus PTTransmCU_In/49  "TCU GearboxIn10"
  S-Function/50 -> CreateBus TCU GearboxIn11/1(In)
  CreateBus TCU GearboxIn11/1(Out) -> CreateBus PTTransmCU_In/50  "TCU GearboxIn11"
  S-Function/51 -> CreateBus TCU GearboxOut0/1(In)
  CreateBus TCU GearboxOut0/1(Out) -> CreateBus PTTransmCU_In/51  "TCU GearboxOut0"
  S-Function/52 -> CreateBus TCU GearboxOut1/1(In)
  CreateBus TCU GearboxOut1/1(Out) -> CreateBus PTTransmCU_In/52  "TCU GearboxOut1"
  S-Function/53 -> CreateBus TCU GearboxOut2/1(In)
  CreateBus TCU GearboxOut2/1(Out) -> CreateBus PTTransmCU_In/53  "TCU GearboxOut2"
  S-Function/54 -> CreateBus TCU GearboxOut3/1(In)
  CreateBus TCU GearboxOut3/1(Out) -> CreateBus PTTransmCU_In/54  "TCU GearboxOut3"
  S-Function/55 -> CreateBus TCU GearboxOut4/1(In)
  CreateBus TCU GearboxOut4/1(Out) -> CreateBus PTTransmCU_In/55  "TCU GearboxOut4"
  S-Function/56 -> CreateBus TCU GearboxOut5/1(In)
  CreateBus TCU GearboxOut5/1(Out) -> CreateBus PTTransmCU_In/56  "TCU GearboxOut5"
  S-Function/57 -> CreateBus TCU GearboxOut6/1(In)
  CreateBus TCU GearboxOut6/1(Out) -> CreateBus PTTransmCU_In/57  "TCU GearboxOut6"
  S-Function/58 -> CreateBus TCU GearboxOut7/1(In)
  CreateBus TCU GearboxOut7/1(Out) -> CreateBus PTTransmCU_In/58  "TCU GearboxOut7"
  S-Function/59 -> CreateBus TCU GearboxOut8/1(In)
  CreateBus TCU GearboxOut8/1(Out) -> CreateBus PTTransmCU_In/59  "TCU GearboxOut8"
  S-Function/60 -> CreateBus TCU GearboxOut9/1(In)
  CreateBus TCU GearboxOut9/1(Out) -> CreateBus PTTransmCU_In/60  "TCU GearboxOut9"
  S-Function/61 -> CreateBus TCU GearboxOut10/1(In)
  CreateBus TCU GearboxOut10/1(Out) -> CreateBus PTTransmCU_In/61  "TCU GearboxOut10"
  S-Function/62 -> CreateBus TCU GearboxOut11/1(In)
  CreateBus TCU GearboxOut11/1(Out) -> CreateBus PTTransmCU_In/62  "TCU GearboxOut11"
  CreateBus TCU ClutchIn0/1(Out) -> CreateBus PTTransmCU_In/15  "TCU ClutchIn0"

== system generic_src/CarMaker/IPG Vehicle/PowerTrain/TCU Example/PTTransmCU_Out ==
  TCU Status : Inport
  TCU ClutchOut : Inport  Port=2
  TCU GearboxOut : Inport  Port=3
  Bus Selector1 : BusSelector  OutputSignals=TCU GearboxOut0,TCU GearboxOut1,TCU GearboxOut2,TCU GearboxOut3,TCU GearboxOut4,TCU GearboxOut5,TCU GearboxOut6,TCU GearboxOut7,TCU GearboxOut8,TCU GearboxOut9,TCU GearboxOut10,TCU GearboxOut11
  Bus Selector2 : BusSelector  OutputSignals=TCU ClutchOut0,TCU ClutchOut1,TCU ClutchOut2,TCU ClutchOut3,TCU ClutchOut4,TCU ClutchOut5,TCU ClutchOut6,TCU ClutchOut7,TCU ClutchOut8,TCU ClutchOut9,TCU ClutchOut10,TCU ClutchOut11
  S-Function : S-Function  FunctionName=cm_pttransmcu_out  SFunctionDeploymentMode=off  EnableBusSupport=off
  wires:
  TCU Status/1 -> S-Function/1
  TCU ClutchOut/1 -> Bus Selector2/1
  Bus Selector2/1 -> S-Function/2  "<TCU ClutchOut0>"
  Bus Selector2/2 -> S-Function/3  "<TCU ClutchOut1>"
  Bus Selector2/3 -> S-Function/4  "<TCU ClutchOut2>"
  Bus Selector2/4 -> S-Function/5  "<TCU ClutchOut3>"
  Bus Selector2/5 -> S-Function/6  "<TCU ClutchOut4>"
  Bus Selector2/6 -> S-Function/7  "<TCU ClutchOut5>"
  Bus Selector2/7 -> S-Function/8  "<TCU ClutchOut6>"
  Bus Selector2/8 -> S-Function/9  "<TCU ClutchOut7>"
  Bus Selector2/9 -> S-Function/10  "<TCU ClutchOut8>"
  Bus Selector2/10 -> S-Function/11  "<TCU ClutchOut9>"
  Bus Selector2/11 -> S-Function/12  "<TCU ClutchOut10>"
  Bus Selector2/12 -> S-Function/13  "<TCU ClutchOut11>"
  TCU GearboxOut/1 -> Bus Selector1/1
  Bus Selector1/1 -> S-Function/14  "<TCU GearboxOut0>"
  Bus Selector1/2 -> S-Function/15  "<TCU GearboxOut1>"
  Bus Selector1/3 -> S-Function/16  "<TCU GearboxOut2>"
  Bus Selector1/4 -> S-Function/17  "<TCU GearboxOut3>"
  Bus Selector1/5 -> S-Function/18  "<TCU GearboxOut4>"
  Bus Selector1/6 -> S-Function/19  "<TCU GearboxOut5>"
  Bus Selector1/7 -> S-Function/20  "<TCU GearboxOut6>"
  Bus Selector1/8 -> S-Function/21  "<TCU GearboxOut7>"
  Bus Selector1/9 -> S-Function/22  "<TCU GearboxOut8>"
  Bus Selector1/10 -> S-Function/23  "<TCU GearboxOut9>"
  Bus Selector1/11 -> S-Function/24  "<TCU GearboxOut10>"
  Bus Selector1/12 -> S-Function/25  "<TCU GearboxOut11>"

== system generic_src/CarMaker/IPG Vehicle/PowerTrain/TCU Example/TCU ClutchOut ==
  BusCreator : BusCreator  Inputs=12
  CreateBus TCU ClutchOut0 : Subsystem
  CreateBus TCU ClutchOut1 : Subsystem
  CreateBus TCU ClutchOut10 : Subsystem
  CreateBus TCU ClutchOut11 : Subsystem
  CreateBus TCU ClutchOut2 : Subsystem
  CreateBus TCU ClutchOut3 : Subsystem
  CreateBus TCU ClutchOut4 : Subsystem
  CreateBus TCU ClutchOut5 : Subsystem
  CreateBus TCU ClutchOut6 : Subsystem
  CreateBus TCU ClutchOut7 : Subsystem
  CreateBus TCU ClutchOut8 : Subsystem
  CreateBus TCU ClutchOut9 : Subsystem
  Ground TCU ClutchOut{1..12} (12 alike) : Ground
  TCU ClutchOut0 : Outport
  wires:
  Ground TCU ClutchOut5/1 -> CreateBus TCU ClutchOut2/1(In)
  Ground TCU ClutchOut6/1 -> CreateBus TCU ClutchOut3/1(In)
  Ground TCU ClutchOut3/1 -> CreateBus TCU ClutchOut0/1(In)
  CreateBus TCU ClutchOut0/1(Out) -> BusCreator/1  "TCU ClutchOut0"
  CreateBus TCU ClutchOut1/1(Out) -> BusCreator/2  "TCU ClutchOut1"
  CreateBus TCU ClutchOut2/1(Out) -> BusCreator/3  "TCU ClutchOut2"
  CreateBus TCU ClutchOut3/1(Out) -> BusCreator/4  "TCU ClutchOut3"
  Ground TCU ClutchOut1/1 -> CreateBus TCU ClutchOut4/1(In)
  CreateBus TCU ClutchOut4/1(Out) -> BusCreator/5  "TCU ClutchOut4"
  Ground TCU ClutchOut2/1 -> CreateBus TCU ClutchOut5/1(In)
  Ground TCU ClutchOut7/1 -> CreateBus TCU ClutchOut1/1(In)
  Ground TCU ClutchOut4/1 -> CreateBus TCU ClutchOut6/1(In)
  CreateBus TCU ClutchOut5/1(Out) -> BusCreator/6  "TCU ClutchOut5"
  CreateBus TCU ClutchOut6/1(Out) -> BusCreator/7  "TCU ClutchOut6"
  Ground TCU ClutchOut8/1 -> CreateBus TCU ClutchOut7/1(In)
  CreateBus TCU ClutchOut7/1(Out) -> BusCreator/8  "TCU ClutchOut7"
  Ground TCU ClutchOut9/1 -> CreateBus TCU ClutchOut8/1(In)
  CreateBus TCU ClutchOut8/1(Out) -> BusCreator/9  "TCU ClutchOut8"
  Ground TCU ClutchOut10/1 -> CreateBus TCU ClutchOut9/1(In)
  CreateBus TCU ClutchOut9/1(Out) -> BusCreator/10  "TCU ClutchOut9"
  Ground TCU ClutchOut11/1 -> CreateBus TCU ClutchOut10/1(In)
  CreateBus TCU ClutchOut10/1(Out) -> BusCreator/11  "TCU ClutchOut10"
  Ground TCU ClutchOut12/1 -> CreateBus TCU ClutchOut11/1(In)
  CreateBus TCU ClutchOut11/1(Out) -> BusCreator/12  "TCU ClutchOut11"
  BusCreator/1 -> TCU ClutchOut0/1  "TCU ClutchOut"

== system generic_src/CarMaker/IPG Vehicle/PowerTrain/TCU Example/TCU Example ==
  note: Shifting Table containing the rot.velocity
      | and gear number for up- and downshift
      | e.g.:
      | MyModel.GearShift:
      |     1    2000    4500
      |     2    2000    4500
      |     3    2000    4500
      |     4    2000    4500
      |     5    2000    5000
  note: this simple model doesn't use the
      | Lock-up functionality of the converter clutch
  Ignition : Inport
  Gearbox : Inport  Port=2
  GearboxIn.GearNo : Inport  Port=3
  Clutch_rotv_out : Inport  Port=4
  SelectorCtrl : Inport  Port=5
  Gearbox.nFGear : Inport  Port=6
  Gearbox.nBGear : Inport  Port=7
  lastGearNoTrg : Inport  Port=8
  Bus Creator : BusCreator  Inputs=2
  Bus Creator1 : BusCreator  Inputs=2
  Bus Selector : BusSelector  OutputSignals=TCU GearboxOut0 set_ParkBrake
  Bus Selector1 : BusSelector  OutputSignals=TCU GearboxIn0 GearNoTrg,TCU GearboxIn0 set_ParkBrake
  Bus Selector2 : BusSelector  OutputSignals=TCU GearboxOut0 GearNoTrg
  Calculate GearNoTrg : Subsystem  TreatAsAtomicUnit=on
  Constant : Constant
  Constant1 : Constant
  Ignition On? : Switch  Criteria=u2 ~= 0
  Limit GearNoTrg : Subsystem
  NOTSET : simulink/Logic and Bit Operations/Compare To Constant  relop===  const=-99999  OutDataTypeStr=uint8
  Read CM Parameter : CarMaker4SL/Read CM Parameter  xfile=Vehicle  xkey=MyModel.GearShift  xnout=80  xdefaults=0  xmuxed=on  xstime=Continuous
      settings: SourceProductName=CarMaker4SL
  Retrun Zero : Subsystem  TreatAsAtomicUnit=on
  Switch : Switch  Criteria=u2 ~= 0
  if Parkposition set 'set_ParkBrake' to 1 : Switch  Criteria=u2 ~= 0
  GearNoTrg : Outport  VectorParamsAs1DForOutWhenUnconnected=off
  set_ParkBrake : Outport  Port=2  VectorParamsAs1DForOutWhenUnconnected=off
  ClutchPos : Outport  Port=3  VectorParamsAs1DForOutWhenUnconnected=off
  wires:
  Constant1/1 -> if Parkposition set 'set_ParkBrake' to 1/3
  Bus Selector/1 -> if Parkposition set 'set_ParkBrake' to 1/1  "<TCU GearboxOut0 set_ParkBrake>"
  if Parkposition set 'set_ParkBrake' to 1/1 -> Bus Creator1/2  "TCU GearboxIn0 set_ParkBrake"
  Retrun Zero/1(GearboxOut) -> Ignition On?/3
  Bus Selector1/2 -> set_ParkBrake/1  "<TCU GearboxIn0 set_ParkBrake>"
  Bus Selector1/1 -> GearNoTrg/1  "<TCU GearboxIn0 GearNoTrg>"
  Gearbox.nBGear/1 -> Bus Creator/2
  lastGearNoTrg/1 -> Calculate GearNoTrg/4(lastGearNoTrg)
  Limit GearNoTrg/1(GearNoTrg_limited) -> Switch/3
  Calculate GearNoTrg/1(GearNoTrg) -> Switch/1  "GearNoTrg"
  Switch/1 -> Bus Creator1/1  "TCU GearboxIn0 GearNoTrg"
  Bus Creator1/1 -> Ignition On?/1
  Read CM Parameter/1 -> Calculate GearNoTrg/5(ShiftingTable)
  SelectorCtrl/1 -> if Parkposition set 'set_ParkBrake' to 1/2, Calculate GearNoTrg/3(SelectorCtrl)
  Clutch_rotv_out/1 -> Calculate GearNoTrg/2(rotvRef)
  Ignition/1 -> Ignition On?/2
  Bus Creator/1 -> Limit GearNoTrg/2(nGears)
  Bus Selector2/1 -> NOTSET/1, Limit GearNoTrg/1(GearNoTrg)  "<TCU GearboxOut0 GearNoTrg>"
  NOTSET/1 -> Switch/2
  Constant/1 -> ClutchPos/1  "Gearbox Clutch Pos"
  GearboxIn.GearNo/1 -> Calculate GearNoTrg/1(GearNo)
  Gearbox.nFGear/1 -> Calculate GearNoTrg/6(nFGears), Bus Creator/1
  Gearbox/1 -> Bus Selector2/1, Bus Selector/1
  Ignition On?/1 -> Bus Selector1/1

== system generic_src/CarMaker/IPG Vehicle/PowerTrain/TCU Example/TCU GearboxOut ==
  In1 : Inport
  In2 : Inport  Port=2
  In3 : Inport  Port=3
  In4 : Inport  Port=4
  Bus Assignment : BusAssignment  AssignedSignals=TCU GearboxOut0 GearNoTrg,TCU GearboxOut0 set_ParkBrake,TCU GearboxOut0 Clutch Pos,TCU GearboxOut0 Trq_DriveSrc_trg
  BusCreator : BusCreator  Inputs=12
  CreateBus TCU GearboxOut0 : Subsystem
  CreateBus TCU GearboxOut1 : Subsystem
  CreateBus TCU GearboxOut10 : Subsystem
  CreateBus TCU GearboxOut11 : Subsystem
  CreateBus TCU GearboxOut2 : Subsystem
  CreateBus TCU GearboxOut3 : Subsystem
  CreateBus TCU GearboxOut4 : Subsystem
  CreateBus TCU GearboxOut5 : Subsystem
  CreateBus TCU GearboxOut6 : Subsystem
  CreateBus TCU GearboxOut7 : Subsystem
  CreateBus TCU GearboxOut8 : Subsystem
  CreateBus TCU GearboxOut9 : Subsystem
  Ground TCU GearboxOut{0..11} (12 alike) : Ground
  TCU GearboxOut : Outport
  wires:
  In1/1 -> Bus Assignment/2
  In2/1 -> Bus Assignment/3
  Ground TCU GearboxOut0/1 -> CreateBus TCU GearboxOut0/1(In)
  CreateBus TCU GearboxOut0/1(Out) -> Bus Assignment/1
  Ground TCU GearboxOut2/1 -> CreateBus TCU GearboxOut2/1(In)
  Ground TCU GearboxOut1/1 -> CreateBus TCU GearboxOut1/1(In)
  Ground TCU GearboxOut3/1 -> CreateBus TCU GearboxOut3/1(In)
  In3/1 -> Bus Assignment/4
  In4/1 -> Bus Assignment/5
  Bus Assignment/1 -> BusCreator/1  "TCU GearboxOut0"
  CreateBus TCU GearboxOut1/1(Out) -> BusCreator/2  "TCU GearboxOut1"
  CreateBus TCU GearboxOut2/1(Out) -> BusCreator/3  "TCU GearboxOut2"
  CreateBus TCU GearboxOut3/1(Out) -> BusCreator/4  "TCU GearboxOut3"
  Ground TCU GearboxOut4/1 -> CreateBus TCU GearboxOut4/1(In)
  CreateBus TCU GearboxOut4/1(Out) -> BusCreator/5  "TCU GearboxOut4"
  Ground TCU GearboxOut5/1 -> CreateBus TCU GearboxOut5/1(In)
  CreateBus TCU GearboxOut5/1(Out) -> BusCreator/6  "TCU GearboxOut5"
  CreateBus TCU GearboxOut6/1(Out) -> BusCreator/7  "TCU GearboxOut6"
  Ground TCU GearboxOut6/1 -> CreateBus TCU GearboxOut6/1(In)
  CreateBus TCU GearboxOut7/1(Out) -> BusCreator/8  "TCU GearboxOut7"
  Ground TCU GearboxOut7/1 -> CreateBus TCU GearboxOut7/1(In)
  Ground TCU GearboxOut8/1 -> CreateBus TCU GearboxOut8/1(In)
  CreateBus TCU GearboxOut8/1(Out) -> BusCreator/9  "TCU GearboxOut8"
  Ground TCU GearboxOut9/1 -> CreateBus TCU GearboxOut9/1(In)
  CreateBus TCU GearboxOut9/1(Out) -> BusCreator/10  "TCU GearboxOut9"
  CreateBus TCU GearboxOut10/1(Out) -> BusCreator/11  "TCU GearboxOut10"
  Ground TCU GearboxOut10/1 -> CreateBus TCU GearboxOut10/1(In)
  CreateBus TCU GearboxOut11/1(Out) -> BusCreator/12  "TCU GearboxOut11"
  Ground TCU GearboxOut11/1 -> CreateBus TCU GearboxOut11/1(In)
  BusCreator/1 -> TCU GearboxOut/1  "TCU GearBoxOut"

== system generic_src/CarMaker/IPG Vehicle/Brake/HydBrakeCU Example/ESP Controller/ESP General System ==
  ESP Input Signals : Inport
  User Input Signals : Inport  Port=2
  Vehicle Input Params : Inport  Port=3
  Ideal_In : Inport  Port=4
  ABS : Subsystem
  ASR : Subsystem
  Bus Creator : BusCreator  Inputs=7
  Bus Creator2 : BusCreator  Inputs=5
  Bus Creator3 : BusCreator  Inputs=6
  Bus Creator4 : BusCreator  Inputs=4
  ESP : Subsystem
  HSA : Subsystem
  Master Controller : Subsystem
  Signal Handling : Subsystem
  ESP Out : Outport  VectorParamsAs1DForOutWhenUnconnected=off
  wires:
  Bus Creator/1 -> ESP Out/1
  ESP Input Signals/1 -> Signal Handling/1(ESP In)
  ESP/1(ESP On) -> Master Controller/2(ESP On)  "ESP On"
  ESP/2(Pilot Valves) -> Bus Creator2/1  "Pilot Valves"
  ESP/3(Suction Valves) -> Bus Creator2/2  "Suction Valves"
  ESP/4(Brake Valves) -> Bus Creator2/3  "Brake Valves"
  ESP/5(Pump Ctrl) -> Bus Creator2/4  "Pump Ctrl"
  ESP/6(Gas_Out) -> Bus Creator2/5  "Gas_Out"
  Bus Creator2/1 -> Master Controller/3(ESP Bus)  "ESP Bus"
  ASR/1(ASR On) -> Master Controller/4(ASR On)  "ASR On"
  ABS/1(ABS On) -> Master Controller/6(ABS On)  "ABS On"
  Bus Creator3/1 -> Master Controller/5(ASR Bus)  "ASR Bus"
  Master Controller/1(ECU Flags) -> Bus Creator/1  "ECU Flags"
  Master Controller/2(Brake Valves) -> Bus Creator/2  "Brake Valves"
  Master Controller/3(Pilot Valves) -> Bus Creator/3  "Pilot Valves"
  Master Controller/4(Suction Valves) -> Bus Creator/4  "Suction Valves"
  Master Controller/5(Pump Ctrl) -> Bus Creator/5  "Pump Ctrl"
  ASR/2(Pilot Valves) -> Bus Creator3/1  "Pilot Valves"
  ASR/3(Suction Valves) -> Bus Creator3/2  "Suction Valves"
  ASR/4(Brake Valves) -> Bus Creator3/3  "Brake Valves"
  ASR/5(Pump Ctrl) -> Bus Creator3/4  "Pump Ctrl"
  ASR/6(Gas_out) -> Bus Creator3/5  "Gas_Out"
  ABS/2(Pilot Valves) -> Bus Creator4/1  "Pilot Valves"
  ABS/3(Suction Valves) -> Bus Creator4/2  "Suction Valves"
  ABS/4(Brake Valves) -> Bus Creator4/3  "Brake Valves"
  ABS/5(Pump Ctrl) -> Bus Creator4/4  "Pump Ctrl"
  Bus Creator4/1 -> Master Controller/7(ABS Bus)  "ABS Bus"
  User Input Signals/1 -> Master Controller/10(User In), ESP/4(User_In), ASR/4(User_In), ABS/4(User_In)
  Vehicle Input Params/1 -> Signal Handling/2(Vehicle Params), ESP/3(Vehicle Params), ASR/3(Vehicle Params), ABS/3(Vehicle Params)
  ASR/7(Diff_Torque) -> Bus Creator3/6  "Diff_Torque"
  Master Controller/6(Diff_Torque) -> Bus Creator/6  "Diff_Torque"
  Ideal_In/1 -> HSA/2(Ideal_In), ABS/2(Ideal_In), ESP/2(Ideal_In), ASR/2(Ideal_In)
  Master Controller/7(VC_Out) -> Bus Creator/7  "VC_Out"
  Signal Handling/2(Signal Bus ESP) -> ESP/1(ESP Signal Bus)
  Signal Handling/3(Signal Bus ASR) -> ASR/1(ASR Signal Bus)
  Signal Handling/4(Signal Bus ABS) -> ABS/1(ABS Signal Bus)
  Signal Handling/5(Signal Bus HSA) -> HSA/1(HSA Signal Bus)
  HSA/1(HSA On) -> Master Controller/8(HSA On)
  HSA/2(BrakePark_Out) -> Master Controller/9(HSA Bus)  "BrakePark"
  Signal Handling/1(Signal Bus Master Controller) -> Master Controller/1(Signal In)
